simulink model "test_identificazione"  (R2025b)
settings: Solver=VariableStepAuto  StartTime=0.0  StopTime=20  RelTol=1e-3
undefined symbols (not defined in the file): imp_amp_d, imp_dur_d, sin_amp_u, sin_frq_u, stp_amp_d, stp_amp_u, stp_tim_d, stp_tim_u
libraries: cstblocks x4
settings Model: Creator=USER  LastModifiedBy=francesco
settings SolverCC: AlgebraicLoopSolver=TrustRegion
settings DebuggingCC: AlgebraicLoopMsg=none  UnconnectedInputMsg=warning  UnconnectedLineMsg=warning
settings ModelReferenceCC: EnableRefExpFcnMdlSchedulingChecks=on
settings RTWCC: GPUComputeCapability=3.5  DLArmComputeVersion=19.05

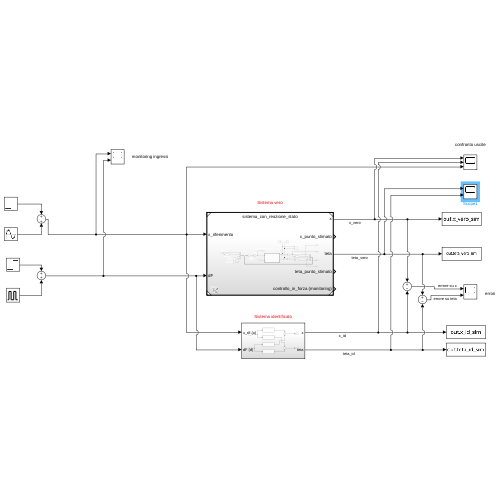
[thumbnail: Simulink's stored preview of the top-level diagram]
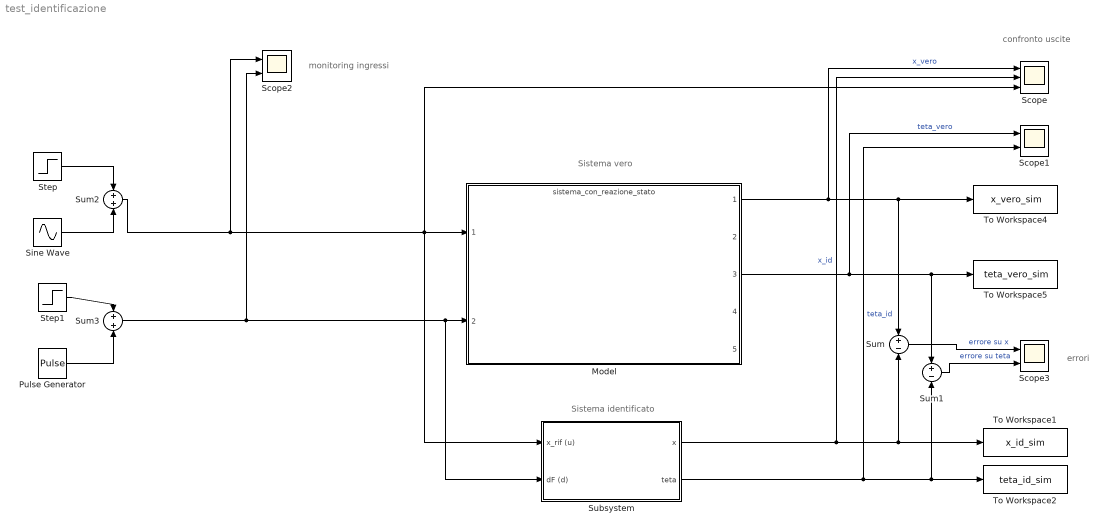
== system test_identificazione ==
  note: monitoring ingressi
  note: confronto uscite
  note: errori
  note: Sistema vero
  note: Sistema identificato
  Model : ModelReference  ModelNameDialog=sistema_con_reazione_stato.slx  SimulationMode=Normal  ModelReferenceVersion=9.55
  Pulse Generator : DiscretePulseGenerator  PulseType=Time based  Amplitude=imp_amp_d  Period=1000  PulseWidth=imp_dur_d / 1000 * 100
  Scope : Scope  NumInputPorts=3
      settings: ActiveDisplayYMinimum=-2.6617021041719275  ActiveDisplayYMaximum=0.30834081141002062
  Scope1 : Scope  NumInputPorts=2
      settings: ActiveDisplayYMinimum=-0.32518065393489937  ActiveDisplayYMaximum=0.14983849326569948
  Scope2 : Scope  NumInputPorts=2
      settings: ActiveDisplayYMinimum=-1  ActiveDisplayYMaximum=1  DataLoggingVariableName=ScopeData2
  Scope3 : Scope  NumInputPorts=2
      settings: ActiveDisplayYMinimum=-0.19747097621270088  ActiveDisplayYMaximum=0.071812722286333883  DataLoggingVariableName=ScopeData3
  Sine Wave : Sin  Amplitude=sin_amp_u  Frequency=sin_frq_u  SampleTime=0
  Step : Step  Time=stp_tim_u  After=stp_amp_u  SampleTime=0
  Step1 : Step  Time=stp_tim_d  After=stp_amp_d  SampleTime=0
  Subsystem : Subsystem
  Sum : Sum  Inputs=+|-
  Sum1 : Sum  Inputs=+|-
  Sum2 : Sum
  Sum3 : Sum
  To Workspace1 : ToWorkspace  VariableName=x_id_sim  SaveFormat=Timeseries  SampleTime=-1
  To Workspace2 : ToWorkspace  VariableName=teta_id_sim  SaveFormat=Timeseries  SampleTime=-1
  To Workspace4 : ToWorkspace  VariableName=x_vero_sim  SaveFormat=Timeseries  SampleTime=-1
  To Workspace5 : ToWorkspace  VariableName=teta_vero_sim  SaveFormat=Timeseries  SampleTime=-1
  wires:
  Model/1 -> Scope/1, To Workspace4/1, Sum/1  "x_vero"
  Model/3 -> Scope1/1, Sum1/1, To Workspace5/1  "teta_vero"
  Subsystem/1(x) -> Scope/2, Sum/2, To Workspace1/1  "x_id"
  Subsystem/2(teta) -> Scope1/2, Sum1/2, To Workspace2/1  "teta_id"
  Sum3/1 -> Model/2, Subsystem/2(dF (d)), Scope2/2
  Sum2/1 -> Subsystem/1(x_rif (u)), Model/1, Scope/3, Scope2/1
  Step/1 -> Sum2/1
  Sine Wave/1 -> Sum2/2
  Sum/1 -> Scope3/1  "errore su x"
  Sum1/1 -> Scope3/2  "errore su teta"
  Step1/1 -> Sum3/1
  Pulse Generator/1 -> Sum3/2

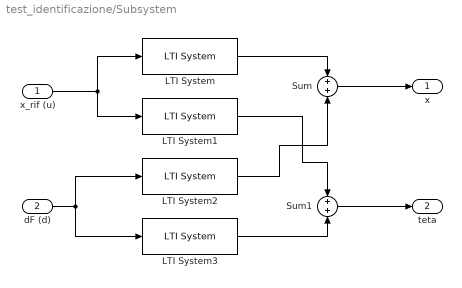
== system test_identificazione/Subsystem ==
  x_rif (u) : Inport
  dF (d) : Inport  Port=2
  LTI System : cstblocks/LTI System  sys=G_u_x  IC=[]  PadeOrder=0
  LTI System1 : cstblocks/LTI System  sys=G_u_teta  IC=[]  PadeOrder=0
  LTI System2 : cstblocks/LTI System  sys=G_d_x  IC=[]  PadeOrder=0
  LTI System3 : cstblocks/LTI System  sys=G_d_teta  IC=[]  PadeOrder=0
  Sum : Sum  Inputs=+|+
  Sum1 : Sum  Inputs=+|+
  x : Outport
  teta : Outport  Port=2
  wires:
  x_rif (u)/1 -> LTI System1/1, LTI System/1
  dF (d)/1 -> LTI System2/1, LTI System3/1
  LTI System/1 -> Sum/1
  Sum/1 -> x/1
  LTI System3/1 -> Sum1/2
  Sum1/1 -> teta/1
  LTI System2/1 -> Sum/2
  LTI System1/1 -> Sum1/1
